simulink model "rtwdemo_preprocessor_subsys"  (Simulink 7.6)
settings: Solver=FixedStepDiscrete  StartTime=0.0  StopTime=100  FixedStep=1  RelTol=1e-3
PostLoadFcn:
  | load rtwdemo_preprocessor_data.mat
Description:
  | Code Variants Using Subsystems
settings Model: Creator=The MathWorks Inc.
settings DataIOCC: SaveFormat=StructureWithTime
settings OptimizationCC: InlineParams=on  InlineInvariantSignals=on  StrengthReduction=on  PassReuseOutputArgsAs=Individual arguments  ZeroExternalMemoryAtStartup=off  ZeroInternalMemoryAtStartup=off  OptimizeModelRefInitCode=on  LifeSpan=1
settings DebuggingCC: MergeDetectMultiDrivingBlocksExec=error  UniqueDataStoreMsg=error  ModelReferenceSymbolNameMessage=none  StrictBusMsg=ErrorOnBusTreatedAsVector
settings HardwareCC: ProdIntDivRoundTo=Zero  ProdEndianess=LittleEndian  ProdHWDeviceType=Generic->32-bit Embedded Processor
settings ModelReferenceCC: ModelReferencePassRootInputsByReference=off
settings RTWCC: SystemTargetFile=ert.tlc  TemplateMakefile=ert_default_tmf  Description=Real-Time Workshop Embedded Coder  GenerateReport=on  RTWVerbose=off  ProcessScript=ert_make_rtw_hook  IncludeHyperlinkInReport=on  LaunchReport=on
settings CodeAppCC: IgnoreCustomStorageClasses=off  IgnoreTestpoints=on
settings ERTTargetCC: MultiwordLength=2048  GenerateSampleERTMain=on  SupportNonFinite=off  InlinedParameterPlacement=NonHierarchical  ERTCustomFileTemplate=example_file_process.tlc  ERTFilePackagingFormat=CompactWithDataFile  ConvertIfToSwitch=off

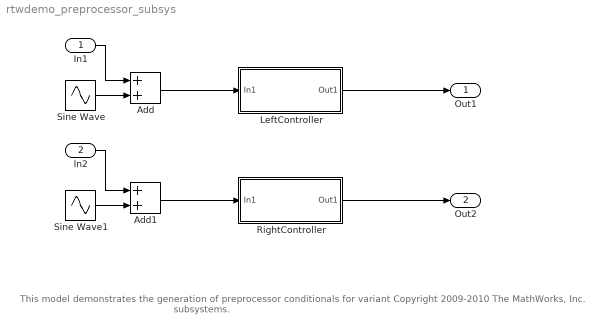
== system rtwdemo_preprocessor_subsys ==
  note: This model demonstrates the generation of
      | preprocessor conditionals for variant subsystems.
  note: Copyright 2009-2010 The MathWorks, Inc.
  In1 : Inport  OutDataTypeStr=double  PortDimensions=1  SampleTime=1
  In2 : Inport  Port=2  OutDataTypeStr=double  PortDimensions=1  SampleTime=1
  Add : Sum
  Add1 : Sum
  LeftController : Subsystem  Variant=on
      settings: GeneratePreprocessorConditionals=on
  RightController : Subsystem  Variant=on
      settings: GeneratePreprocessorConditionals=on
  Sine Wave : Sin  SineType=Sample based  Samples=40  SampleTime=1
  Sine Wave1 : Sin  SineType=Sample based  Samples=40  SampleTime=1  Offset=20
  Out1 : Outport  OutDataTypeStr=double  PortDimensions=1  SampleTime=1
  Out2 : Outport  Port=2  OutDataTypeStr=double  PortDimensions=1  SampleTime=1
  wires:
  Add/1 -> LeftController/1(In1)
  LeftController/1(Out1) -> Out1/1
  Add1/1 -> RightController/1(In1)
  RightController/1(Out1) -> Out2/1
  In1/1 -> Add/1
  Sine Wave/1 -> Add/2
  In2/1 -> Add1/1
  Sine Wave1/1 -> Add1/2

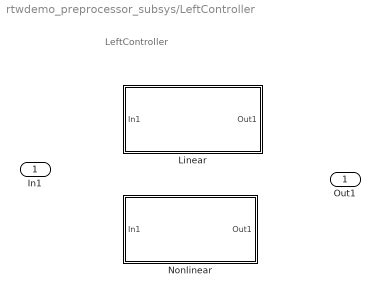
== system rtwdemo_preprocessor_subsys/LeftController ==
  note: LeftController
  In1 : Inport
  Linear : Subsystem  TreatAsAtomicUnit=on  VariantObject=LINEAR
  Nonlinear : Subsystem  TreatAsAtomicUnit=on  VariantObject=NONLINEAR
  Out1 : Outport

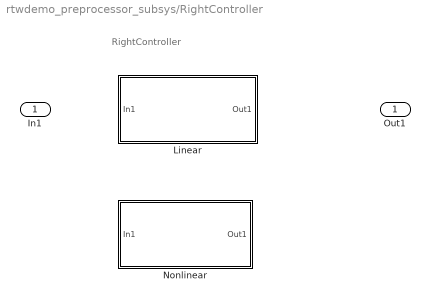
== system rtwdemo_preprocessor_subsys/RightController ==
  note: RightController
  In1 : Inport
  Linear : Subsystem  TreatAsAtomicUnit=on  VariantObject=LINEAR
  Nonlinear : Subsystem  TreatAsAtomicUnit=on  VariantObject=NONLINEAR
  Out1 : Outport

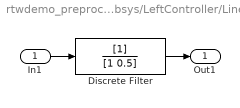
== system rtwdemo_preprocessor_subsys/LeftController/Linear ==
  In1 : Inport
  Discrete Filter : DiscreteFilter
  Out1 : Outport
  wires:
  Discrete Filter/1 -> Out1/1
  In1/1 -> Discrete Filter/1

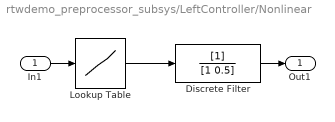
== system rtwdemo_preprocessor_subsys/LeftController/Nonlinear ==
  In1 : Inport
  Discrete Filter : DiscreteFilter
  Lookup Table : Lookup  InputValues=[-1 -0.5 0 0.5 1]  Table=[-1 0 0 0 1]
  Out1 : Outport
  wires:
  In1/1 -> Lookup Table/1
  Discrete Filter/1 -> Out1/1
  Lookup Table/1 -> Discrete Filter/1

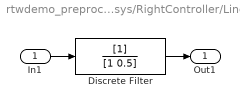
== system rtwdemo_preprocessor_subsys/RightController/Linear ==
  In1 : Inport
  Discrete Filter : DiscreteFilter
  Out1 : Outport
  wires:
  In1/1 -> Discrete Filter/1
  Discrete Filter/1 -> Out1/1

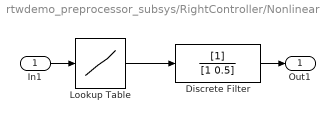
== system rtwdemo_preprocessor_subsys/RightController/Nonlinear ==
  In1 : Inport
  Discrete Filter : DiscreteFilter
  Lookup Table : Lookup  InputValues=[-1 -0.5 0 0.5 1]  Table=[-1 0 0 0 1]
  Out1 : Outport
  wires:
  Lookup Table/1 -> Discrete Filter/1
  Discrete Filter/1 -> Out1/1
  In1/1 -> Lookup Table/1
